simulink model "six_dof_custom"  (R2026a)
settings: Solver=VariableStepAuto
values from neighbouring files (symbols this model uses):
  I = [ 0.0093, 0, 0 ... (first row only)    [dz_3_model.m]    (also in six_dof_eq.m = [Ixx, Ixy, Ixz)
  mass_quadrotor = 1.07    [dz_3_model.m]
settings Model: Creator=vas77  LastModifiedBy=vas77

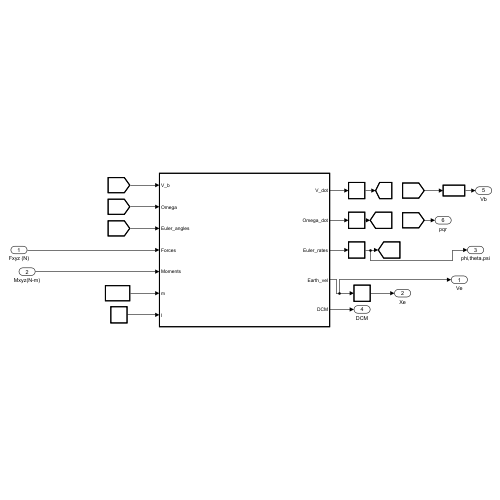
[thumbnail: Simulink's stored preview of the top-level diagram]
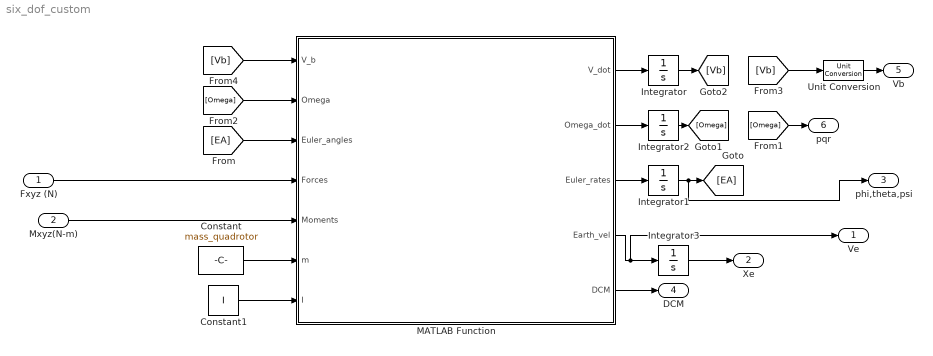
== system six_dof_custom ==
  Fxyz (N) : Inport  PortDimensions=3
  Mxyz(N-m) : Inport  Port=2  PortDimensions=3
  Constant : Constant  Value=mass_quadrotor
  Constant1 : Constant  Value=I
  Integrator{,1..3} (4 alike) : Integrator  InitialCondition=[0; 0; 0]
  MATLAB Function : MATLAB Function  TreatAsAtomicUnit=on
  Unit Conversion : UnitConversion
  Ve : Outport  PortDimensions=3
  Xe : Outport  Port=2
  phi,theta,psi : Outport  Port=3
  DCM : Outport  Port=4
  Vb : Outport  Port=5
  pqr : Outport  Port=6
  wires:
  Fxyz (N)/1 -> MATLAB Function/4(Forces)
  Constant/1 -> MATLAB Function/6(m)
  MATLAB Function/1(V_dot) -> Integrator/1
  Unit Conversion/1 -> Vb/1
  MATLAB Function/3(Euler_rates) -> Integrator1/1
  Mxyz(N-m)/1 -> MATLAB Function/5(Moments)
  Constant1/1 -> MATLAB Function/7(I)
  MATLAB Function/2(Omega_dot) -> Integrator2/1
  MATLAB Function/4(Earth_vel) -> Ve/1, Integrator3/1
  Integrator3/1 -> Xe/1
  [EA] -> MATLAB Function/3(Euler_angles)
  [Omega] -> pqr/1
  Integrator2/1 -> [Omega]
  [Omega] -> MATLAB Function/2(Omega)
  [Vb] -> Unit Conversion/1
  Integrator/1 -> [Vb]
  [Vb] -> MATLAB Function/1(V_b)
  MATLAB Function/5(DCM) -> DCM/1
  Integrator1/1 -> phi,theta,psi/1, [EA]

== matlab function six_dof_custom/MATLAB Function ==
  data: V_b input; V_dot output; Omega_dot output; Omega input; Euler_angles input; Forces input; Moments input; m input; Euler_rates output; I input; Earth_vel output; DCM output
function [V_dot, Omega_dot, Euler_rates, Earth_vel, DCM] = full_drone_model(V_b, Omega, Euler_angles, Forces, Moments, m, I)
    % Force all incoming signals to be column vectors
    V_b = V_b(:);
    Omega = Omega(:);
    Euler_angles = Euler_angles(:);
    Forces = Forces(:);
    Moments = Moments(:);

    % Unpack angles
    phi = Euler_angles(1);
    theta = Euler_angles(2);
    psi = Euler_angles(3);

    % 1. Translational Dynamics (Body Accelerations)
    % V_dot = F/m - (Omega x V_b)
    V_dot = (Forces / m) - cross(Omega, V_b);

    % 2. Rotational Dynamics (Angular Accelerations)
    % Omega_dot = I^-1 * (M - Omega x (I*Omega))
    % Note: In MATLAB, inv(I) computes the inverse of the Inertia matrix
    Omega_dot = inv(I) * (Moments - cross(Omega, I * Omega));

    % 3. Rotational Kinematics (Euler Angle Rates)
    H = [1, sin(phi)*tan(theta), cos(phi)*tan(theta);
         0, cos(phi),           -sin(phi);
         0, sin(phi)/cos(theta), cos(phi)/cos(theta)];
         
    Euler_rates = H * Omega;

    % 4. Translational Kinematics (Earth-Relative Velocities)
    % The Direction Cosine Matrix (DCM) for standard Yaw-Pitch-Roll sequence
    DCM = [cos(theta)*cos(psi), sin(phi)*sin(theta)*cos(psi) - cos(phi)*sin(psi), cos(phi)*sin(theta)*cos(psi) + sin(phi)*sin(psi);
           cos(theta)*sin(psi), sin(phi)*sin(theta)*sin(psi) + cos(phi)*cos(psi), cos(phi)*sin(theta)*sin(psi) - sin(phi)*cos(psi);
          -sin(theta),          sin(phi)*cos(theta),                              cos(phi)*cos(theta)];
          
    Earth_vel = DCM * V_b;
end
